simulink model "vacuum_object"  (R2023a)
settings: Solver=FixedStepDiscrete  StartTime=0.0  StopTime=inf  FixedStep=0.001  RelTol=1e-3  EnableMultiTasking=on
PreLoadFcn:
  | frs = FrankaRobotSettings;
undefined symbols (not defined in the file): FrankaVacuumGripperControlModes
libraries: franka_simulink_library x4, simulink x2
settings Model: SimulationMode=external  ExtModeTrigDuration=10000  Creator=vasi_ko  LastModifiedBy=kvasios
settings SolverCC: AlgebraicLoopSolver=TrustRegion
settings DataIOCC: LimitDataPoints=on  SaveFormat=Array  ReturnWorkspaceOutputs=off
settings OptimizationCC: EnhancedBackFolding=on  PassReuseOutputArgsThreshold=0  OptimizeBlockOrder=speed  DifferentSizesBufferReuse=on  OptimizationCustomize=off
settings DebuggingCC: SolverPrmCheckMsg=warning  ParameterTunabilityLossMsg=error  UnconnectedInputMsg=warning  UnconnectedOutputMsg=warning  UnconnectedLineMsg=warning  SFUnexpectedBacktrackingDiag=warning  SFNoUnconditionalDefaultTransitionDiag=warning  SFExecutionAtInitializationDiag=none  ArithmeticOperatorsInVariantConditions=warning
settings ModelReferenceCC: EnableRefExpFcnMdlSchedulingChecks=on  PropagateSignalLabelsOutOfModel=off
settings SFSimCC: SimUseLocalCustomCode=off  MATLABDynamicMemAlloc=off  CustomCodeUndefinedFunction=UseInterfaceOnly  SimTargetLang=C++
settings RTWCC: RTWVerbose=off  RTWUseLocalCustomCode=off  BuildConfiguration=Faster Runs  TargetLang=C++  DLArmComputeVersion=19.05
settings CodeAppCC: ForceParamTrailComments=on  OperatorAnnotations=on
settings ConfigComp: CovMetricSettings=dw  CovSaveCumulativeToWorkspaceVar=on  CovSaveSingleToWorkspaceVar=on  CovExternalEMLEnable=off  CovSFcnEnable=off

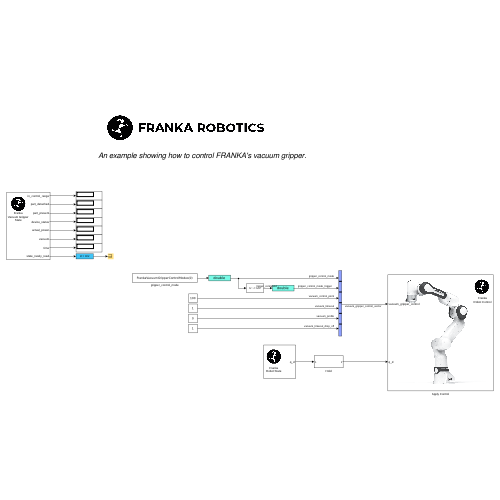
[thumbnail: Simulink's stored preview of the top-level diagram]
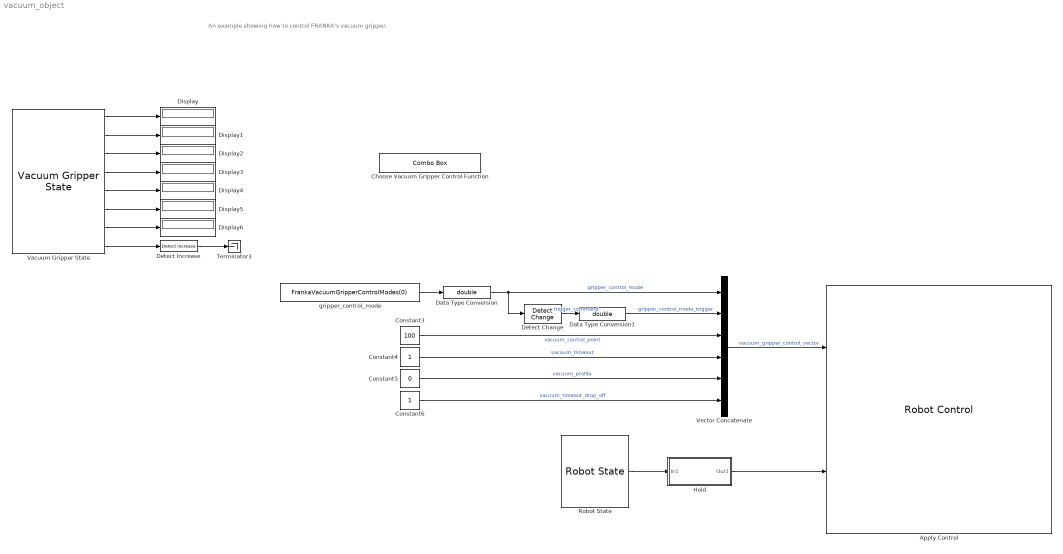
== system vacuum_object ==
  note: An example showing how to control FRANKA's vacuum gripper.
  Apply Control : franka_simulink_library/Robot Control  robot_ip=frs.robot_ip  gripper_selection=Franka Vacuum Gripper  control_mode=Joint Positions - Internal Controller Mode  controller_choice=Joint Impedance Controller  joint_impedance=frs.joint_impedance_stiffness  cartesian_impedance=[3000, 3000, 3000, 300, 300, 300]  rate_limiter=on  cuttoff_frequency=frs.cutoff_frequency  elbow_control=off  collision_thresholds=frs.collision_thresholds.getAs1DArray  load_inertia=frs.load_inertia.getAs1DArray  NE_T_EE=frs.NE_T_EE(:)  EE_T_K=frs.EE_T_K(:)  init_joint_configuration_req=on  init_joint_configuration=frs.home_configuration
      settings: SourceProductName=Franka Robotics Simulink Support Package
  Choose Vacuum Gripper Control Function : ComboBox  LabelPosition=Bottom  SelectedLabel=idle  UseEnumeratedDataType=on  EnumeratedDataType=FrankaVacuumGripperControlModes
      settings: Values={{'idle', 'read_state', 'vacuum', 'dropOff', 'stop'}, [0 1 2 3 4]}
  Constant3 : Constant  Value=100
  Constant4 : Constant
  Constant5 : Constant  Value=0
  Constant6 : Constant
  Data Type Conversion : DataTypeConversion  OutDataTypeStr=double  SaturateOnIntegerOverflow=off  RndMeth=Floor
  Data Type Conversion1 : DataTypeConversion  OutDataTypeStr=double  SaturateOnIntegerOverflow=off  RndMeth=Floor
  Detect Change : simulink/Logic and Bit Operations/Detect Change  vinit=0  OutDataTypeStr=boolean
  Detect Increase : simulink/Logic and Bit Operations/Detect Increase  vinit=0.0  OutDataTypeStr=boolean
  Display{,1..6} (7 alike) : Display
  Hold : Subsystem
  Robot State : franka_simulink_library/Robot State  robot_ip=frs.robot_ip  signals_requested='q_d'
      settings: SourceProductName=Franka Robotics Simulink Support Package
  Terminator3 : Terminator
  Vacuum Gripper State : franka_simulink_library/Vacuum Gripper State  robot_ip=frs.robot_ip
      settings: SourceProductName=Franka Robotics Simulink Support Package
  Vector Concatenate : Concatenate  NumInputs=6
  gripper_control_mode : Constant  Value=FrankaVacuumGripperControlModes(0)  SampleTime=-1
  wires:
  Detect Increase/1 -> Terminator3/1
  Vacuum Gripper State/8 -> Detect Increase/1
  gripper_control_mode/1 -> Data Type Conversion/1
  Vacuum Gripper State/1 -> Display/1
  Vacuum Gripper State/7 -> Display6/1
  Vector Concatenate/1 -> Apply Control/1  "vacuum_gripper_control_vector"
  Data Type Conversion/1 -> Detect Change/1, Vector Concatenate/1  "gripper_control_mode"
  Constant3/1 -> Vector Concatenate/3  "vacuum_control_point"
  Constant4/1 -> Vector Concatenate/4  "vacuum_timeout"
  Constant5/1 -> Vector Concatenate/5  "vacuum_profile"
  Constant6/1 -> Vector Concatenate/6  "vacuum_timeout_drop_off"
  Detect Change/1 -> Data Type Conversion1/1  "trigger_command"
  Robot State/1 -> Hold/1(In1)
  Hold/1(Out1) -> Apply Control/2
  Vacuum Gripper State/2 -> Display1/1
  Vacuum Gripper State/3 -> Display2/1
  Vacuum Gripper State/4 -> Display3/1
  Vacuum Gripper State/5 -> Display4/1
  Vacuum Gripper State/6 -> Display5/1
  Data Type Conversion1/1 -> Vector Concatenate/2  "gripper_control_mode_trigger"

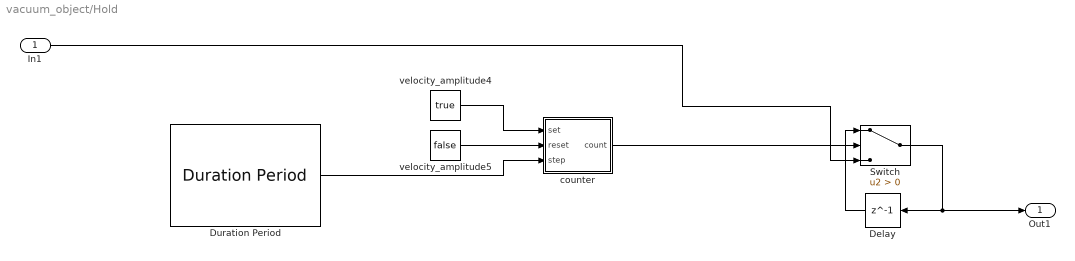
== system vacuum_object/Hold ==
  In1 : Inport
  Delay : Delay  DelayLength=1
  Duration Period : franka_simulink_library/Duration Period  robot_ip=frs.robot_ip
      settings: SourceProductName=Franka Robotics Simulink Support Package
  Switch : Switch  Criteria=u2 > Threshold  SaturateOnIntegerOverflow=off  InputSameDT=off
  counter : Subsystem
  velocity_amplitude4 : Constant  Value=true  VectorParams1D=off
  velocity_amplitude5 : Constant  Value=false  VectorParams1D=off
  Out1 : Outport
  wires:
  counter/1(count) -> Switch/2
  velocity_amplitude4/1 -> counter/1(set)
  velocity_amplitude5/1 -> counter/2(reset)
  In1/1 -> Switch/3
  Delay/1 -> Switch/1
  Switch/1 -> Out1/1, Delay/1
  Duration Period/1 -> counter/3(step)

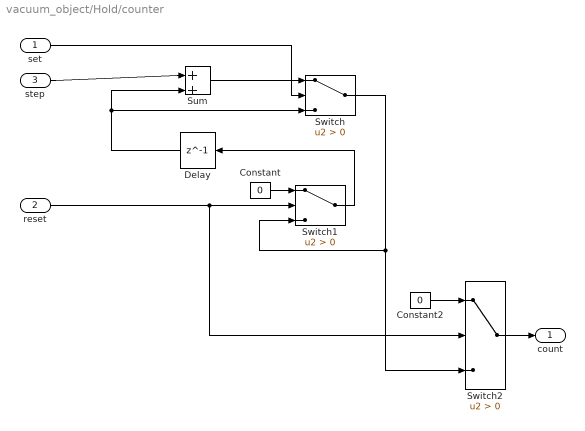
== system vacuum_object/Hold/counter ==
  set : Inport  OutDataTypeStr=boolean
  reset : Inport  Port=2  OutDataTypeStr=boolean
  step : Inport  Port=3  OutDataTypeStr=double
  Constant : Constant  Value=0  OutDataTypeStr=double
  Constant2 : Constant  Value=0  OutDataTypeStr=double
  Delay : Delay  DelayLength=1  InitialCondition=0
  Sum : Sum  Inputs=|++
  Switch : Switch  Criteria=u2 > Threshold  SaturateOnIntegerOverflow=off  InputSameDT=off
  Switch1 : Switch  Criteria=u2 > Threshold  OutDataTypeStr=double  SaturateOnIntegerOverflow=off  InputSameDT=off
  Switch2 : Switch  Criteria=u2 > Threshold  OutDataTypeStr=double  SaturateOnIntegerOverflow=off  InputSameDT=off
  count : Outport  OutDataTypeStr=double  VectorParamsAs1DForOutWhenUnconnected=off
  wires:
  Switch2/1 -> count/1
  Constant2/1 -> Switch2/1
  Sum/1 -> Switch/1
  set/1 -> Switch/2
  Switch/1 -> Switch1/3, Switch2/3
  step/1 -> Sum/1
  Delay/1 -> Sum/2, Switch/3
  reset/1 -> Switch1/2, Switch2/2
  Constant/1 -> Switch1/1
  Switch1/1 -> Delay/1
